simulink model "test_libMdl_TrainFrontDataGenerator"  (R2018a)
settings: Solver=FixedStepDiscrete  StartTime=0  StopTime=t_end  RelTol=1e-3
PreLoadFcn:
  | init_test_libMdl_TrainFrontDataGenerator
InitFcn:
  | init_test_libMdl_TrainFrontDataGenerator
values from neighbouring files (symbols this model uses):
  a_train_0 = 0    [init_test_libMdl_TrainFrontDataGenerator.m]
  v_train_0 = v_train_desired_kmh/3.6    (= 55.5555555556)    [init_test_libMdl_TrainFrontDataGenerator.m]
  v_train_desired_kmh = 200    [init_test_libMdl_TrainFrontDataGenerator.m]
libraries: libMdl_TrainFrontDataGenerator x1
settings Model: SimulationMode=accelerator  PauseTimes=224  Creator=hwinter  LastModifiedBy=Hanno
settings DataIOCC: SaveOutput=off  SignalLogging=off  DSMLogging=off  SaveTime=off
settings DebuggingCC: ReadBeforeWriteMsg=DisableAll  WriteAfterWriteMsg=DisableAll  WriteAfterReadMsg=DisableAll  MultiTaskDSMMsg=none
settings HardwareCC: ProdBitPerLong=64  ProdHWDeviceType=Intel->x86-64 (Linux 64)  TargetBitPerPointer=64  TargetBitPerSizeT=64  TargetBitPerPtrDiffT=64  TargetLongLongMode=on  TargetIntDivRoundTo=Zero  TargetEndianess=LittleEndian  TargetWordSize=64  TargetHWDeviceType=MATLAB Host  ProdEqTarget=off
settings SFSimCC: SFSimEcho=off
settings RTWCC: SystemTargetFile=rsim.tlc  TemplateMakefile=rsim_default_tmf  Description=Rapid Simulation Target
settings CodeAppCC: StateflowObjectComments=on
settings RSimTargetCC: TargetLangStandard=C99 (ISO)  GeneratePreprocessorConditionals=Use local settings

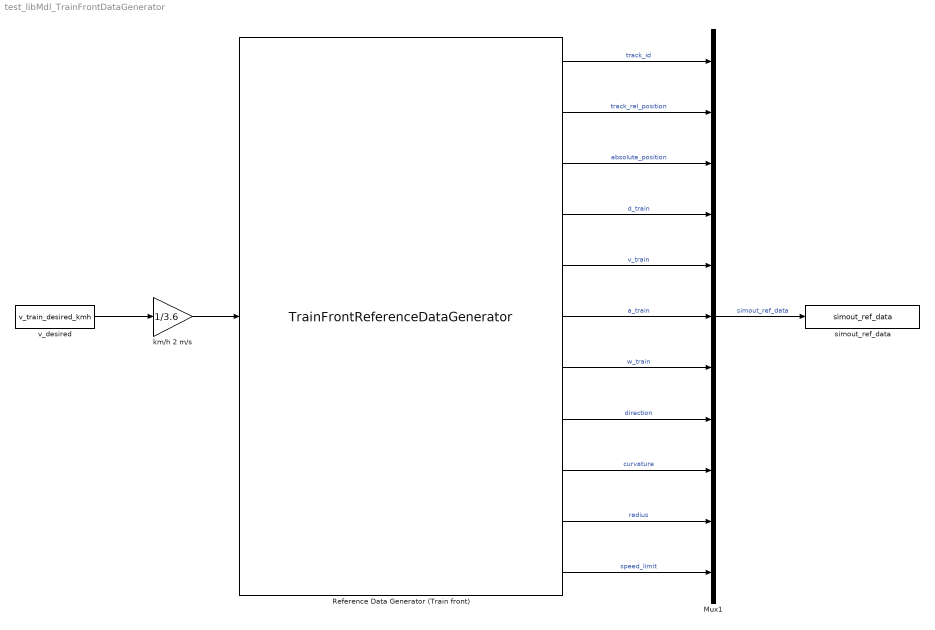
== system test_libMdl_TrainFrontDataGenerator ==
  Mux1 : Mux  Inputs=11
  Reference Data Generator (Train front) : libMdl_TrainFrontDataGenerator/TrainFrontReferenceDataGenerator  mv_T_ref_system=T_system  mv_motion_t_constant=1  mv_a_train_limits=max_train_acc  mv_track_id_0=track_id_0  mv_track_rel_position_0=track_rel_position_0  mv_x_0=[v_train_0, a_train_0]  mv_track_map=mat_track_map  mv_track_map_rot_angle=phi_track
  km/h 2 m/s : Gain  Gain=1/3.6
  simout_ref_data : ToWorkspace  VariableName=simout_ref_data  SaveFormat=Timeseries  SampleTime=-1
  v_desired : Constant  Value=v_train_desired_kmh
  wires:
  v_desired/1 -> km/h 2 m/s/1
  Reference Data Generator (Train front)/6 -> Mux1/6  "a_train"
  Reference Data Generator (Train front)/7 -> Mux1/7  "w_train"
  Reference Data Generator (Train front)/3 -> Mux1/3  "absolute_position"
  km/h 2 m/s/1 -> Reference Data Generator (Train front)/1
  Reference Data Generator (Train front)/11 -> Mux1/11  "speed_limit"
  Reference Data Generator (Train front)/10 -> Mux1/10  "radius"
  Reference Data Generator (Train front)/9 -> Mux1/9  "curvature"
  Reference Data Generator (Train front)/8 -> Mux1/8  "direction"
  Reference Data Generator (Train front)/5 -> Mux1/5  "v_train"
  Reference Data Generator (Train front)/4 -> Mux1/4  "d_train"
  Reference Data Generator (Train front)/2 -> Mux1/2  "track_rel_position"
  Reference Data Generator (Train front)/1 -> Mux1/1  "track_id"
  Mux1/1 -> simout_ref_data/1  "simout_ref_data"
